simulink model "DCM_Integrated_AllModes"  (R2022a)
settings: Solver=FixedStepAuto  StartTime=0.0  StopTime=10.0  FixedStep=1e-3  RelTol=1e-3  EnableMultiTasking=on
undefined symbols (not defined in the file): A0, A1, D0, D1, D10, D11, D12, D13, D2, D3, D4, D5, D6, D7, D8, D9, PTA0, PTA1, PTA2, PTB2, PTB23, PTB3, PTB9, PTC16, PTC17, PTC2, PTC3, PTC4, PTD0, PTD1, PTD2, PTD3
libraries: frdmk64flib x18, etargetslib x6
settings Model: ExtModeTrigDuration=5  Creator=bmile  LastModifiedBy=bmile
settings OptimizationCC: EnhancedBackFolding=on  PassReuseOutputArgsAs=Individual arguments  ZeroExternalMemoryAtStartup=off  ZeroInternalMemoryAtStartup=off  MaxStackSize=64  OptimizeBlockOrder=speed  DifferentSizesBufferReuse=on  OptimizationCustomize=off  EfficientTunableParamExpr=on
settings DebuggingCC: ParameterTunabilityLossMsg=error
settings HardwareCC: ProdBitPerPointer=32  ProdBitPerSizeT=32  ProdBitPerPtrDiffT=32  ProdLargestAtomicInteger=Long  ProdLargestAtomicFloat=Double  ProdWordSize=32  ProdHWDeviceType=ARM Compatible->ARM Cortex
settings SFSimCC: MATLABDynamicMemAlloc=off
settings RTWCC: SystemTargetFile=ert.tlc  HardwareBoard=NXP FRDM-K64F  TLCOptions="-aInlineSetEventsForThisBaseRateFcn=TLC_FALSE -aSuppressMultiTaskScheduler=TLC_FALSE  -aRateBasedStepFcn=0"  TemplateMakefile=ert_default_tmf  Toolchain=GNU Tools for ARM Embedded Processors
settings CodeAppCC: ForceParamTrailComments=on  IgnoreCustomStorageClasses=off  OperatorAnnotations=on  SimulinkDataObjDesc=on  SFDataObjDesc=on  InsertBlockDesc=on
settings ERTTargetCC: ExtModeTransport=4  ExtModeMexFile=sendToCommService

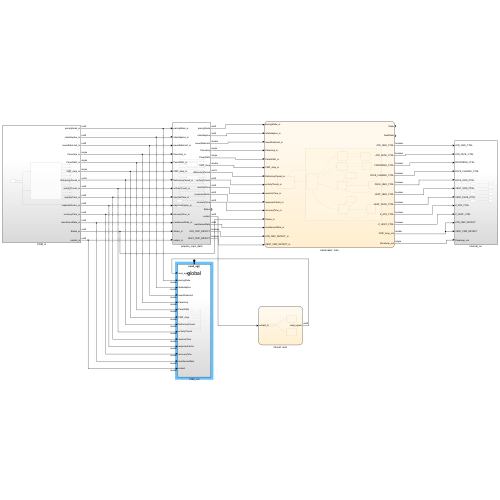
[thumbnail: Simulink's stored preview of the top-level diagram]
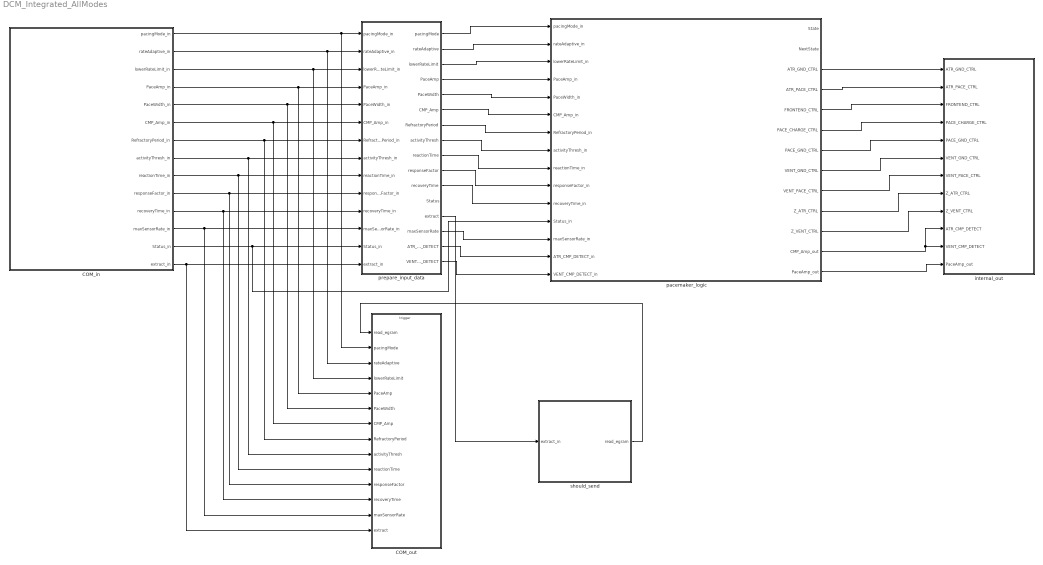
== system DCM_Integrated_AllModes ==
  COM_in : Subsystem
  COM_out : Subsystem
  internal_out : Subsystem
  pacemaker_logic : Stateflow chart  TreatAsAtomicUnit=on
      settings: PortSchema="{\"entries\":[{\"content\":{\"sides\":[{\"content\":{\"connectorIds\":[\"In10\",\"In14\",\"In8\",\"In3\",\"In4\",\"In2\",\"In5\",\"In7\",\"In11\",\"In13\",\"In12\",\"In15\",\"In9\",\"In1\",\"In6\"]},\"type\":\"ConnectorPlacement.EquallySpacedRectSide\",\"uuid\":\"5755a581-9f62-44fc-9995-0c59b8d9bd26\"},{\"content\":{\"connectorIds\":[\"Out7\",\"Out10\",\"Out13\",\"Out12\",\"Out11\",\"Out9\",\"Out8\",\"Out6\",\"Out5\",\"Out4\",\"Out3\",\"Out1\",\"Out2\"],\"side\":\"RIGHT\"},\"type\":\"ConnectorPlacement.EquallySpacedRectSide\",\"uuid\":\"6039a3f0-4c46-4c8e-a591-8e56fd020917\"},{\"content\":{\"connectorIds\":[],\"side\":\"TOP\"},\"type\":\"ConnectorPlacement.EquallySpacedRectSide\",\"uuid\":\"6166557d-37e2-4e7a-805b-c7dff50c5fe9\"}]},\"type\":\"ConnectorPlacement.EquallySpacedConnector\",\"uuid\":\"b44d46a1-ecce-4b19-9699-9237155b3373\"}],\"packageUris\":[\"http://schema.mathworks.com/mf0/Connector/R2020b\"],\"version\":\"1.0\"}"
  prepare_input_data : Subsystem
  should_send : Stateflow chart  TreatAsAtomicUnit=on
  wires:
  COM_in/14(extract_in) -> COM_out/14(extract), prepare_input_data/14(extract_in)
  COM_in/1(pacingMode_in) -> COM_out/2(pacingMode), prepare_input_data/1(pacingMode_in)
  COM_in/2(rateAdaptive_in) -> COM_out/3(rateAdaptive), prepare_input_data/2(rateAdaptive_in)
  COM_in/3(lowerRateLimit_in) -> COM_out/4(lowerRateLimit), prepare_input_data/3(lowerRateLimit_in)
  COM_in/4(PaceAmp_in) -> COM_out/5(PaceAmp), prepare_input_data/4(PaceAmp_in)
  COM_in/5(PaceWidth_in) -> COM_out/6(PaceWidth), prepare_input_data/5(PaceWidth_in)
  COM_in/6(CMP_Amp_in) -> COM_out/7(CMP_Amp), prepare_input_data/6(CMP_Amp_in)
  COM_in/7(RefractoryPeriod_in) -> COM_out/8(RefractoryPeriod), prepare_input_data/7(RefractoryPeriod_in)
  COM_in/8(activityThresh_in) -> COM_out/9(activityThresh), prepare_input_data/8(activityThresh_in)
  COM_in/9(reactionTime_in) -> COM_out/10(reactionTime), prepare_input_data/9(reactionTime_in)
  COM_in/10(responseFactor_in) -> COM_out/11(responseFactor), prepare_input_data/10(responseFactor_in)
  COM_in/11(recoveryTime_in) -> COM_out/12(recoveryTime), prepare_input_data/11(recoveryTime_in)
  COM_in/12(maxSensorRate_in) -> COM_out/13(maxSensorRate), prepare_input_data/12(maxSensorRate_in)
  COM_in/13(Status_in) -> pacemaker_logic/15(Status_in), prepare_input_data/13(Status_in)
  prepare_input_data/1(pacingMode) -> pacemaker_logic/10(pacingMode_in)
  prepare_input_data/2(rateAdaptive) -> pacemaker_logic/14(rateAdaptive_in)
  prepare_input_data/3(lowerRateLimit) -> pacemaker_logic/8(lowerRateLimit_in)
  prepare_input_data/4(PaceAmp) -> pacemaker_logic/3(PaceAmp_in)
  prepare_input_data/5(PaceWidth) -> pacemaker_logic/4(PaceWidth_in)
  prepare_input_data/6(CMP_Amp) -> pacemaker_logic/2(CMP_Amp_in)
  prepare_input_data/7(RefractoryPeriod) -> pacemaker_logic/5(RefractoryPeriod_in)
  prepare_input_data/8(activityThresh) -> pacemaker_logic/7(activityThresh_in)
  prepare_input_data/9(reactionTime) -> pacemaker_logic/11(reactionTime_in)
  prepare_input_data/10(responseFactor) -> pacemaker_logic/13(responseFactor_in)
  prepare_input_data/11(recoveryTime) -> pacemaker_logic/12(recoveryTime_in)
  prepare_input_data/14(maxSensorRate) -> pacemaker_logic/9(maxSensorRate_in)
  prepare_input_data/15(ATR_CMP_DETECT) -> pacemaker_logic/1(ATR_CMP_DETECT_in)
  prepare_input_data/16(VENT_CMP_DETECT) -> pacemaker_logic/6(VENT_CMP_DETECT_in)
  pacemaker_logic/13(ATR_GND_CTRL) -> internal_out/1(ATR_GND_CTRL)
  pacemaker_logic/12(ATR_PACE_CTRL) -> internal_out/2(ATR_PACE_CTRL)
  pacemaker_logic/11(FRONTEND_CTRL) -> internal_out/3(FRONTEND_CTRL)
  pacemaker_logic/8(PACE_GND_CTRL) -> internal_out/5(PACE_GND_CTRL)
  pacemaker_logic/9(PACE_CHARGE_CTRL) -> internal_out/4(PACE_CHARGE_CTRL)
  pacemaker_logic/6(VENT_GND_CTRL) -> internal_out/6(VENT_GND_CTRL)
  pacemaker_logic/5(VENT_PACE_CTRL) -> internal_out/7(VENT_PACE_CTRL)
  pacemaker_logic/4(Z_ATR_CTRL) -> internal_out/8(Z_ATR_CTRL)
  pacemaker_logic/3(Z_VENT_CTRL) -> internal_out/9(Z_VENT_CTRL)
  pacemaker_logic/1(CMP_Amp_out) -> internal_out/11(VENT_CMP_DETECT), internal_out/10(ATR_CMP_DETECT)
  pacemaker_logic/2(PaceAmp_out) -> internal_out/12(PaceAmp_out)
  should_send/1(read_egram) -> COM_out/1(read_egram)
  prepare_input_data/13(extract) -> should_send/1(extract_in)

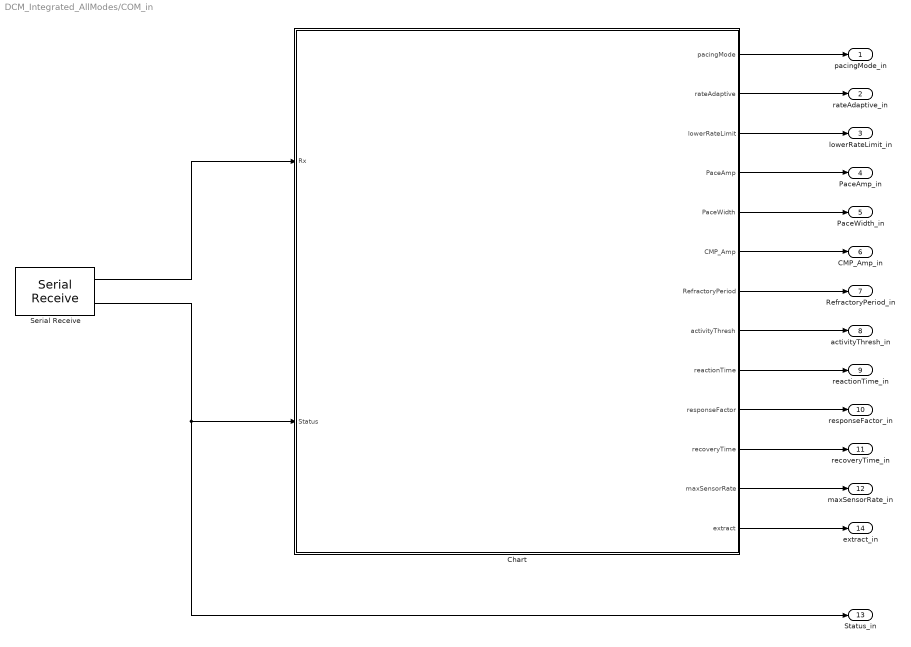
== system DCM_Integrated_AllModes/COM_in ==
  Chart : Stateflow chart  TreatAsAtomicUnit=on
      settings: PortSchema="{\"entries\":[{\"content\":{\"sides\":[{\"content\":{\"connectorIds\":[\"In1\",\"In2\"]},\"type\":\"ConnectorPlacement.EquallySpacedRectSide\",\"uuid\":\"3381abbf-739a-4b97-b1d1-7c6f9c0d83ce\"},{\"content\":{\"connectorIds\":[\"Out9\",\"Out13\",\"Out7\",\"Out2\",\"Out3\",\"Out1\",\"Out4\",\"Out5\",\"Out10\",\"Out12\",\"Out11\",\"Out8\",\"Out6\"],\"side\":\"RIGHT\"},\"type\":\"ConnectorPlacement.EquallySpacedRectSide\",\"uuid\":\"3d52d84e-16e5-42ed-9d61-42c4dbf660e5\"},{\"content\":{\"connectorIds\":[],\"side\":\"TOP\"},\"type\":\"ConnectorPlacement.EquallySpacedRectSide\",\"uuid\":\"6fb9aaab-cc36-471e-9a0e-4b804908c392\"}]},\"type\":\"ConnectorPlacement.EquallySpacedConnector\",\"uuid\":\"d6192154-0e66-4236-86c4-bef785add890\"}],\"packageUris\":[\"http://schema.mathworks.com/mf0/Connector/R2020b\"],\"version\":\"1.0\"}"
  Serial Receive : frdmk64flib/Serial Receive  SCIModule=0  Baudrate=uint32(9600)  Parity=None  StopBits=1  HardwareFlowControl=None  ByteOrder=LittleEndian  DataType=uint8  DataLength=24  BlockingMode=off  OutputStatus=on  SampleTime=0.1
  pacingMode_in : Outport
  rateAdaptive_in : Outport  Port=2
  lowerRateLimit_in : Outport  Port=3
  PaceAmp_in : Outport  Port=4
  PaceWidth_in : Outport  Port=5
  CMP_Amp_in : Outport  Port=6
  RefractoryPeriod_in : Outport  Port=7
  activityThresh_in : Outport  Port=8
  reactionTime_in : Outport  Port=9
  responseFactor_in : Outport  Port=10
  recoveryTime_in : Outport  Port=11
  maxSensorRate_in : Outport  Port=12
  Status_in : Outport  Port=13
  extract_in : Outport  Port=14
  wires:
  Serial Receive/1 -> Chart/1(Rx)
  Serial Receive/2 -> Status_in/1, Chart/2(Status)
  Chart/9(pacingMode) -> pacingMode_in/1
  Chart/13(rateAdaptive) -> rateAdaptive_in/1
  Chart/7(lowerRateLimit) -> lowerRateLimit_in/1
  Chart/2(PaceAmp) -> PaceAmp_in/1
  Chart/3(PaceWidth) -> PaceWidth_in/1
  Chart/1(CMP_Amp) -> CMP_Amp_in/1
  Chart/4(RefractoryPeriod) -> RefractoryPeriod_in/1
  Chart/5(activityThresh) -> activityThresh_in/1
  Chart/10(reactionTime) -> reactionTime_in/1
  Chart/12(responseFactor) -> responseFactor_in/1
  Chart/11(recoveryTime) -> recoveryTime_in/1
  Chart/8(maxSensorRate) -> maxSensorRate_in/1
  Chart/6(extract) -> extract_in/1

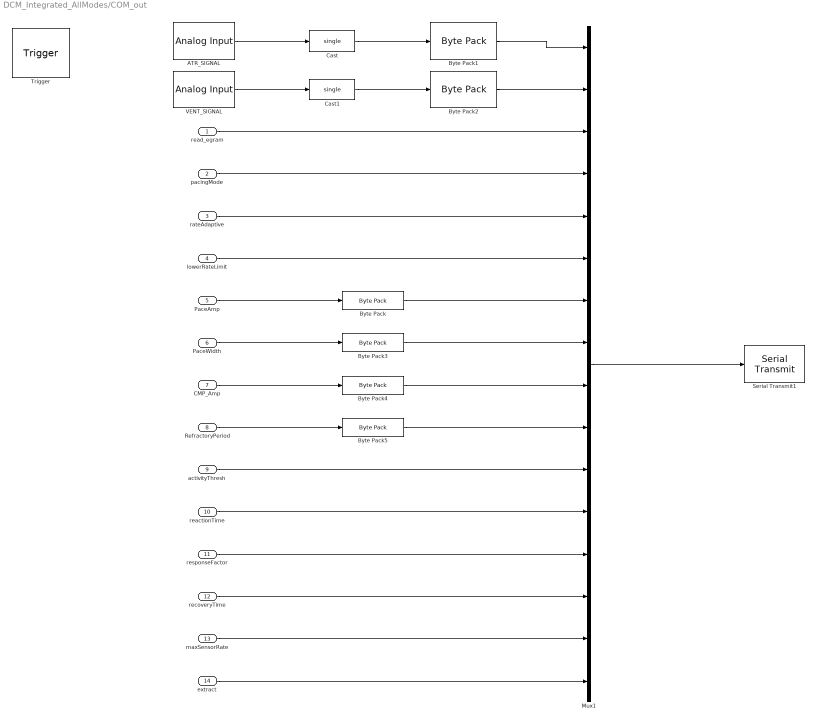
== system DCM_Integrated_AllModes/COM_out ==
  read_egram : Inport
  pacingMode : Inport  Port=2
  rateAdaptive : Inport  Port=3
  lowerRateLimit : Inport  Port=4
  PaceAmp : Inport  Port=5
  PaceWidth : Inport  Port=6
  CMP_Amp : Inport  Port=7
  RefractoryPeriod : Inport  Port=8
  activityThresh : Inport  Port=9
  reactionTime : Inport  Port=10
  responseFactor : Inport  Port=11
  recoveryTime : Inport  Port=12
  maxSensorRate : Inport  Port=13
  extract : Inport  Port=14
  Trigger : TriggerPort  TriggerType=function-call  IsSimulinkFunction=on  FunctionName=send_eg  VariantControl=(inherit)  PortDimensions=1
  ATR_SIGNAL : frdmk64flib/Analog Input  Whichpin=PTB2 (A0)  SampleTime=-1
  Byte Pack{,1..4} (5 alike) : etargetslib/Byte Pack  datatypes={'single'}  byteAlign=1
  Byte Pack5 : etargetslib/Byte Pack  datatypes={'uint16'}  byteAlign=1
  Cast : DataTypeConversion  OutDataTypeStr=single  SaturateOnIntegerOverflow=off  RndMeth=Floor
  Cast1 : DataTypeConversion  OutDataTypeStr=single  SaturateOnIntegerOverflow=off  RndMeth=Floor
  Mux1 : Mux  Inputs=16
  Serial Transmit1 : frdmk64flib/Serial Transmit  SCIModule=0  Baudrate=uint32(9600)  Parity=None  StopBits=1  HardwareFlowControl=None  ByteOrder=LittleEndian  BlockingMode=on  OutputStatus=off
  VENT_SIGNAL : frdmk64flib/Analog Input  Whichpin=PTB3 (A1)  SampleTime=-1
  wires:
  read_egram/1 -> Mux1/3
  Byte Pack1/1 -> Mux1/1
  Byte Pack2/1 -> Mux1/2
  Mux1/1 -> Serial Transmit1/1
  Cast1/1 -> Byte Pack2/1
  VENT_SIGNAL/1 -> Cast1/1
  ATR_SIGNAL/1 -> Cast/1
  Cast/1 -> Byte Pack1/1
  pacingMode/1 -> Mux1/4
  rateAdaptive/1 -> Mux1/5
  lowerRateLimit/1 -> Mux1/6
  extract/1 -> Mux1/16
  maxSensorRate/1 -> Mux1/15
  recoveryTime/1 -> Mux1/14
  responseFactor/1 -> Mux1/13
  reactionTime/1 -> Mux1/12
  activityThresh/1 -> Mux1/11
  PaceAmp/1 -> Byte Pack/1
  PaceWidth/1 -> Byte Pack3/1
  CMP_Amp/1 -> Byte Pack4/1
  Byte Pack4/1 -> Mux1/9
  Byte Pack3/1 -> Mux1/8
  Byte Pack/1 -> Mux1/7
  RefractoryPeriod/1 -> Byte Pack5/1
  Byte Pack5/1 -> Mux1/10

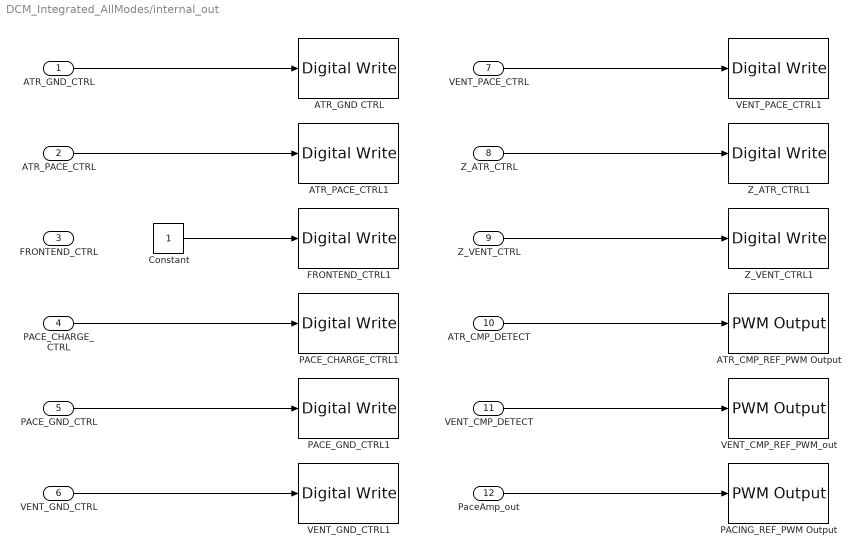
== system DCM_Integrated_AllModes/internal_out ==
  ATR_GND_CTRL : Inport
  ATR_PACE_CTRL : Inport  Port=2
  FRONTEND_CTRL : Inport  Port=3
  PACE_CHARGE_CTRL : Inport  Port=4
  PACE_GND_CTRL : Inport  Port=5
  VENT_GND_CTRL : Inport  Port=6
  VENT_PACE_CTRL : Inport  Port=7
  Z_ATR_CTRL : Inport  Port=8
  Z_VENT_CTRL : Inport  Port=9
  ATR_CMP_DETECT : Inport  Port=10
  VENT_CMP_DETECT : Inport  Port=11
  PaceAmp_out : Inport  Port=12
  ATR_CMP_REF_PWM Output : frdmk64flib/PWM Output  Whichpin=PTC2 (D6)  InitialFrequency=2000  InitialDutyCycle=0
  ATR_GND CTRL : frdmk64flib/Digital Write  Whichpin=PTD2 (D11)
  ATR_PACE_CTRL1 : frdmk64flib/Digital Write  Whichpin=PTA0 (D8)
  Constant : Constant  OutDataTypeStr=boolean
  FRONTEND_CTRL1 : frdmk64flib/Digital Write  Whichpin=PTD1 (D13)
  PACE_CHARGE_CTRL1 : frdmk64flib/Digital Write  Whichpin=PTB9 (D2)
  PACE_GND_CTRL1 : frdmk64flib/Digital Write  Whichpin=PTD0 (D10)
  PACING_REF_PWM Output : frdmk64flib/PWM Output  Whichpin=PTA2 (D5)  InitialFrequency=2000  InitialDutyCycle=0
  VENT_CMP_REF_PWM_out : frdmk64flib/PWM Output  Whichpin=PTA1 (D3)  InitialFrequency=2000  InitialDutyCycle=0
  VENT_GND_CTRL1 : frdmk64flib/Digital Write  Whichpin=PTD3 (D12)
  VENT_PACE_CTRL1 : frdmk64flib/Digital Write  Whichpin=PTC4 (D9)
  Z_ATR_CTRL1 : frdmk64flib/Digital Write  Whichpin=PTB23 (D4)
  Z_VENT_CTRL1 : frdmk64flib/Digital Write  Whichpin=PTC3 (D7)
  wires:
  ATR_GND_CTRL/1 -> ATR_GND CTRL/1
  ATR_PACE_CTRL/1 -> ATR_PACE_CTRL1/1
  PACE_CHARGE_CTRL/1 -> PACE_CHARGE_CTRL1/1
  PACE_GND_CTRL/1 -> PACE_GND_CTRL1/1
  VENT_GND_CTRL/1 -> VENT_GND_CTRL1/1
  PaceAmp_out/1 -> PACING_REF_PWM Output/1
  VENT_CMP_DETECT/1 -> VENT_CMP_REF_PWM_out/1
  ATR_CMP_DETECT/1 -> ATR_CMP_REF_PWM Output/1
  Z_VENT_CTRL/1 -> Z_VENT_CTRL1/1
  Z_ATR_CTRL/1 -> Z_ATR_CTRL1/1
  VENT_PACE_CTRL/1 -> VENT_PACE_CTRL1/1
  Constant/1 -> FRONTEND_CTRL1/1

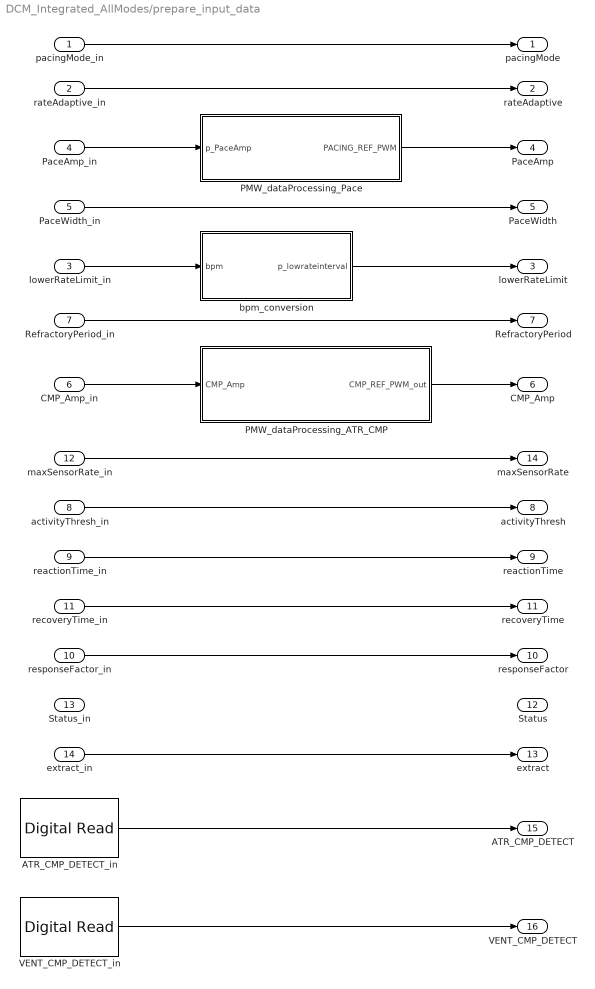
== system DCM_Integrated_AllModes/prepare_input_data ==
  pacingMode_in : Inport
  rateAdaptive_in : Inport  Port=2
  lowerRateLimit_in : Inport  Port=3
  PaceAmp_in : Inport  Port=4
  PaceWidth_in : Inport  Port=5
  CMP_Amp_in : Inport  Port=6
  RefractoryPeriod_in : Inport  Port=7
  activityThresh_in : Inport  Port=8
  reactionTime_in : Inport  Port=9
  responseFactor_in : Inport  Port=10
  recoveryTime_in : Inport  Port=11
  maxSensorRate_in : Inport  Port=12
  Status_in : Inport  Port=13
  extract_in : Inport  Port=14
  ATR_CMP_DETECT_in : frdmk64flib/Digital Read  Whichpin=PTC16 (D0)  SampleTime=-1
  PMW_dataProcessing_ATR_CMP : Subsystem
  PMW_dataProcessing_Pace : Subsystem
  VENT_CMP_DETECT_in : frdmk64flib/Digital Read  Whichpin=PTC17 (D1)  SampleTime=-1
  bpm_conversion : Subsystem
  pacingMode : Outport
  rateAdaptive : Outport  Port=2
  lowerRateLimit : Outport  Port=3
  PaceAmp : Outport  Port=4
  PaceWidth : Outport  Port=5
  CMP_Amp : Outport  Port=6
  RefractoryPeriod : Outport  Port=7
  activityThresh : Outport  Port=8
  reactionTime : Outport  Port=9
  responseFactor : Outport  Port=10
  recoveryTime : Outport  Port=11
  Status : Outport  Port=12
  extract : Outport  Port=13
  maxSensorRate : Outport  Port=14
  ATR_CMP_DETECT : Outport  Port=15
  VENT_CMP_DETECT : Outport  Port=16
  wires:
  lowerRateLimit_in/1 -> bpm_conversion/1(bpm)
  CMP_Amp_in/1 -> PMW_dataProcessing_ATR_CMP/1(CMP_Amp)
  PaceAmp_in/1 -> PMW_dataProcessing_Pace/1(p_PaceAmp)
  VENT_CMP_DETECT_in/1 -> VENT_CMP_DETECT/1
  ATR_CMP_DETECT_in/1 -> ATR_CMP_DETECT/1
  responseFactor_in/1 -> responseFactor/1
  recoveryTime_in/1 -> recoveryTime/1
  reactionTime_in/1 -> reactionTime/1
  activityThresh_in/1 -> activityThresh/1
  maxSensorRate_in/1 -> maxSensorRate/1
  PMW_dataProcessing_ATR_CMP/1(CMP_REF_PWM_out) -> CMP_Amp/1
  RefractoryPeriod_in/1 -> RefractoryPeriod/1
  bpm_conversion/1(p_lowrateinterval) -> lowerRateLimit/1
  PaceWidth_in/1 -> PaceWidth/1
  PMW_dataProcessing_Pace/1(PACING_REF_PWM) -> PaceAmp/1
  pacingMode_in/1 -> pacingMode/1
  extract_in/1 -> extract/1
  rateAdaptive_in/1 -> rateAdaptive/1

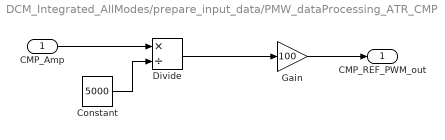
== system DCM_Integrated_AllModes/prepare_input_data/PMW_dataProcessing_ATR_CMP ==
  CMP_Amp : Inport
  Constant : Constant  Value=5000
  Divide : Product  Inputs=*/
  Gain : Gain  Gain=100
  CMP_REF_PWM_out : Outport
  wires:
  Divide/1 -> Gain/1
  Constant/1 -> Divide/2
  CMP_Amp/1 -> Divide/1
  Gain/1 -> CMP_REF_PWM_out/1

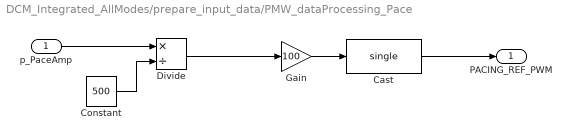
== system DCM_Integrated_AllModes/prepare_input_data/PMW_dataProcessing_Pace ==
  p_PaceAmp : Inport
  Cast : DataTypeConversion  OutDataTypeStr=single  SaturateOnIntegerOverflow=off  RndMeth=Floor
  Constant : Constant  Value=500
  Divide : Product  Inputs=*/
  Gain : Gain  Gain=100
  PACING_REF_PWM : Outport
  wires:
  Divide/1 -> Gain/1
  Constant/1 -> Divide/2
  p_PaceAmp/1 -> Divide/1
  Gain/1 -> Cast/1
  Cast/1 -> PACING_REF_PWM/1

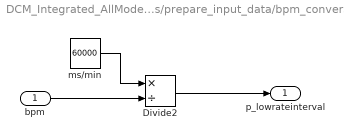
== system DCM_Integrated_AllModes/prepare_input_data/bpm_conversion ==
  bpm : Inport
  Divide2 : Product  Inputs=*/
  ms/min : Constant  Value=60000
  p_lowrateinterval : Outport
  wires:
  ms/min/1 -> Divide2/1
  bpm/1 -> Divide2/2
  Divide2/1 -> p_lowrateinterval/1

== stateflow chart DCM_Integrated_AllModes/COM_in/Chart ==
  state INITIAL
    %Sets initial values of parameters
    entry:
    pacingMode = 1; %uint8; 0-AOO,1-VOO,2-AAI,3-VVI,4-AAIR,5-VVIR
    lowerRateLimit = 60; %uint8; ppm
    maxSensorRate = 120; %uint8; ppm
    PaceAmp = 3.5; %single; V
    PaceWidth = 0; %single; 0-30 ms
    CMP_Amp = 2.5; %single; V
    RefractoryPeriod = 250; %uint16; ms
    activityThresh = 3; %uint8; V-Low,Low,Med-Low,Med,Med-High,High,V-High
    reactionTime = 30; %uint8; s
    responseFactor = 1; %uint8; 1-16
    recoveryTime = 5; %uint8; 2-16 min
    extract = 0; %uint8, denotes data egram data is to be sent to DCM
  state SET_PARAMS
    entry:
    pacingMode = Rx(2);
    rateAdaptive = Rx(3)
    lowerRateLimit = Rx(4);
    PaceAmp = typecast(Rx(5:8), 'single');
    PaceWidth = typecast(Rx(9:12), 'single');
    CMP_Amp = typecast(Rx(13:16), 'single');
    RefractoryPeriod = typecast(Rx(17:18), 'uint16');
    activityThresh = Rx(19);
    reactionTime = Rx(20);
    responseFactor = Rx(21);
    recoveryTime = Rx(22);
    maxSensorRate = Rx(23);
    extract = Rx(24);
  state STANDBY
    %Waits for COM
  (default) -> INITIAL
  (junction 17) -> STANDBY [order 2]
  INITIAL -> STANDBY
  STANDBY -> (junction 17) : [Status == 0]
  (junction 17) -> SET_PARAMS [order 1] : [Rx(1) == 22]
  SET_PARAMS -> STANDBY
  data: Rx input uint8; Status input uint8; CMP_Amp output single; PaceAmp output single; PaceWidth output single; RefractoryPeriod output uint16; activityThresh output uint8; extract output uint8; lowerRateLimit output uint8; maxSensorRate output uint8; pacingMode output uint8; reactionTime output uint8; recoveryTime output uint8; responseFactor output uint8; rateAdaptive output uint8

== stateflow chart DCM_Integrated_AllModes/should_send ==
  state SEND_EGRAM_DATA
    %Sends egram data to DCM
    during:
    read_egram = 1;
    send_eg();
    exit:
    read_egram = 0
    send_eg();
  state IDLE
    %Waits for first extract input
  state DO_NOT_SEND
    %Stops the pacemaker from sending
    %egram data
    entry:
    read_egram = 0;
  IDLE -> SEND_EGRAM_DATA [order 2] : [extract_in == 1]
  (default) -> IDLE
  SEND_EGRAM_DATA -> DO_NOT_SEND : [extract_in == 0]
  DO_NOT_SEND -> SEND_EGRAM_DATA : [extract_in == 1]
  IDLE -> DO_NOT_SEND [order 1] : [extract_in == 0]
  data: extract_in input uint8; read_egram output uint8

== stateflow chart DCM_Integrated_AllModes/pacemaker_logic ==
  state PACEMAKER_WORKING
    %The pacemaker is working in one of the modes in this state
    state AOO_Charging_Discharging
      entry:
      StateTran = false
      NextState = 0
      ATR_PACE_CTRL = false
      VENT_PACE_CTRL=false
      PACE_CHARGE_CTRL = true
      ATR_GND_CTRL = true
      PACE_GND_CTRL = true
      Z_ATR_CTRL=false
      State = 1
      exit:
      StateTran = true
    state AOO_Pace_Heart
      entry:
      StateTran = false
      NextState = 0
      ATR_PACE_CTRL = true
      PACE_CHARGE_CTRL = false
      PACE_GND_CTRL = true
      ATR_GND_CTRL = false
      State = 2
      exit:
      StateTran = true
    state VOO_VENT_Charging_Discharging
      entry:
      NextState = 0
      VENT_PACE_CTRL = false
      ATR_PACE_CTRL = false
      PACE_CHARGE_CTRL = true
      VENT_GND_CTRL = true
      PACE_GND_CTRL = true
      Z_VENT_CTRL=false
      State = 3
      StateTran = false
      exit:
      StateTran = true
    state VOO_VENT_Pace_Heart
      entry:
      NextState = 0
      StateTran = false
      VENT_PACE_CTRL = true
      PACE_CHARGE_CTRL = false
      PACE_GND_CTRL = true
      VENT_GND_CTRL = false
      State = 4
      exit:
      StateTran = true
    state AAI_Pulse_Sensed
      entry:
      NextState = 0
      %FRONTEND_CTRL=false
      State = 6
      StateTran = false
      exit:
      StateTran = true
      wait_time= cast(refract_period,"single")
    state StateOff
      %This state tells the pacemaker which
      %mode it should run, which is decided
      %by ModeOn and is checked on the
      %transistion conditions.
      entry:
      %Initialize all states to 0 or false, since
      %the pacemaker should do nothing in this
      %state.
      StateTran = false
      State = 0
      NextState = 0
      PACE_CHARGE_CTRL = false
      Z_ATR_CTRL = false
      Z_VENT_CTRL = false
      PACE_GND_CTRL = false
      ATR_PACE_CTRL = false
      ATR_GND_CTRL = false
      VENT_GND_CTRL = false
      VENT_PACE_CTRL = false
      FRONTEND_CTRL = false
      exit:
      StateTran = true
      wait_time=pulse_width
    state AAI_Charging_Discharging
      entry:
      NextState = 0
      ATR_PACE_CTRL = false
      VENT_PACE_CTRL=false
      PACE_CHARGE_CTRL = true
      ATR_GND_CTRL = true
      PACE_GND_CTRL = true
      Z_ATR_CTRL=false
      FRONTEND_CTRL=true
      State = 5
      StateTran = false
      exit:
      StateTran = true
    state AAI_Pace_Heart
      entry:
      NextState = 0
      ATR_PACE_CTRL = true
      PACE_CHARGE_CTRL = false
      PACE_GND_CTRL = true
      ATR_GND_CTRL = false
      State = 7
      StateTran = false
      exit:
      StateTran = true
      wait_time=pulse_width
    state VVI_Pulse_Sensed
      entry:
      NextState = 0
      %FRONTEND_CTRL=false
      State = 9
      StateTran = false
      exit:
      StateTran = true
      wait_time= cast(refract_period,"single")
    state VVI_Charging_Discharging
      entry:
      NextState = 0
      ATR_PACE_CTRL = false
      VENT_PACE_CTRL=false
      PACE_CHARGE_CTRL = true
      VENT_GND_CTRL = true
      PACE_GND_CTRL = true
      Z_VENT_CTRL=false
      FRONTEND_CTRL=true
      State = 8
      StateTran = false
      exit:
      StateTran = true
    state VVI_Pace_Heart
      entry:
      NextState = 0
      VENT_PACE_CTRL = true
      PACE_CHARGE_CTRL = false
      PACE_GND_CTRL = true
      VENT_GND_CTRL = false
      State = 10
      StateTran = false
      exit:
      StateTran = true
      wait_time=pulse_width
    AOO_Charging_Discharging -> AOO_Pace_Heart : after(p_lowrateinterval-pulse_width,msec) / {NextState = 2}
    StateOff -> AOO_Charging_Discharging [order 4] : [ModeOn==1] / {NextState = 1}
    AOO_Pace_Heart -> AOO_Charging_Discharging : after(pulse_width,msec) / {NextState = 1}
    VOO_VENT_Charging_Discharging -> VOO_VENT_Pace_Heart : after(p_lowrateinterval-pulse_width,msec) / {NextState = 4}
    VOO_VENT_Pace_Heart -> VOO_VENT_Charging_Discharging : after(pulse_width,msec) / {NextState = 3}
    StateOff -> VOO_VENT_Charging_Discharging [order 3] : [ModeOn==2] / {NextState = 3}
    AAI_Pulse_Sensed -> AAI_Charging_Discharging : [after(refract_period,msec)] / {NextState = 5}
    AAI_Charging_Discharging -> AAI_Pulse_Sensed [order 2] : [ATR_CMP_DETECT == 1] / {NextState = 6}
    StateOff -> AAI_Charging_Discharging [order 1] : [ModeOn==3] / {NextState = 5}
    AAI_Charging_Discharging -> AAI_Pace_Heart [order 1] : [after(p_lowrateinterval-wait_time,msec)] / {NextState = 7}
    AAI_Pace_Heart -> AAI_Charging_Discharging : after(pulse_width,msec) / {NextState = 5}
    StateOff -> VVI_Charging_Discharging [order 2] : [ModeOn==4] / {NextState = 8}
    VVI_Pulse_Sensed -> VVI_Charging_Discharging : [after(refract_period,msec)] / {NextState = 8}
    VVI_Charging_Discharging -> VVI_Pulse_Sensed [order 2] : [VENT_CMP_DETECT == 1] / {NextState = 9}
    VVI_Charging_Discharging -> VVI_Pace_Heart [order 1] : [after(p_lowrateinterval-wait_time,msec)] / {NextState = 10}
    VVI_Pace_Heart -> VVI_Charging_Discharging : after(pulse_width,msec) / {NextState = 8}
  state S_UPDATE_PARAMS
    %This is the state the device takes when it is receiving
    %new data from the DCM
    entry:
    State = 22
    ModeOn = pacingMode_in;
    PaceAmp_out = PaceAmp_in;
    pulse_width = PaceWidth_in;
    p_lowrateinterval = lowerRateLimit_in;
    refract_period = RefractoryPeriod_in;
    ATR_CMP_DETECT = ATR_CMP_DETECT_in;
    VENT_CMP_DETECT = VENT_CMP_DETECT_in;
    CMP_Amp_out = CMP_Amp_in;
    MSR = maxSensorRate_in;
    activityThresh = activityThresh_in;
    recoveryTime = recoveryTime_in;
    reactionTime = reactionTime_in;
    responseFactor = responseFactor_in;
    RA = rateAdaptive_in
  PACEMAKER_WORKING -> S_UPDATE_PARAMS : [Status_in == 0]
  (default) -> S_UPDATE_PARAMS
  S_UPDATE_PARAMS -> StateOff : [Status_in == 32]
  data: ATR_CMP_DETECT_in input; CMP_Amp_in input; PaceAmp_in input; PaceWidth_in input; RefractoryPeriod_in input; VENT_CMP_DETECT_in input; activityThresh_in input; lowerRateLimit_in input; maxSensorRate_in input; pacingMode_in input; reactionTime_in input; recoveryTime_in input; responseFactor_in input; ATR_CMP_DETECT local; CMP_Amp_out output; MSR local; ModeOn local; PaceAmp_out output; VENT_CMP_DETECT local; activityThresh local; p_lowrateinterval local; pulse_width local; reactionTime local; recoveryTime local; refract_period local; responseFactor local; rateAdaptive_in input; wait_time local; Z_VENT_CTRL output; Z_ATR_CTRL output; VENT_PACE_CTRL output; VENT_GND_CTRL output; State output; PACE_GND_CTRL output; PACE_CHARGE_CTRL output; NextState output; FRONTEND_CTRL output; ATR_PACE_CTRL output; ATR_GND_CTRL output; Status_in input; StateTran local; RA local
